simulink model "simu_actuating_fins"  (R2025b)
settings: Solver=FixedStepAuto  StartTime=0.0  StopTime=7  FixedStep=0.01  RelTol=1e-3
model workspace (MAT data in the model file):
  T_data = [16.81; 22.34; 22.23; 21.49; 20; 20.21; 18.09; 15.74; 13.4; 10.85; 10.21; 8.94; 8.83; 8.62; 8.62; 8.62; 8.51; 8.72; 8.51; 8.51; 7.77; 7.02; 5.64; 3.83; 2.23; 0.96; 0]
  aero_data.Alpha = [0; 2; 4]
  aero_data.CD = [0.20580088598; 0.20580088598; 0.20580088598]
  aero_data.CL = [0; 0.0625795358549; 0.124860076206]
  aero_data.CP = [0.999; 0.999; 0.999]
  t_data = [0.01; 0.03; 0.11; 0.26; 0.37; 0.47; 0.67; 0.99; 1.31; 1.81; 2.49; 3.13; 3.6; 4.11; 4.95; 5.45; 5.58; 5.88; 6.22; 6.46; 6.6; 6.71; 6.79; 6.91; 6.95; 7; 7.05]
undefined symbols (not defined in the file): fractalcoef
libraries: mspsensorlib x1, aerolibatmos2 x1, sharedutil x1
settings Model: Creator=arjun  LastModifiedBy=19725

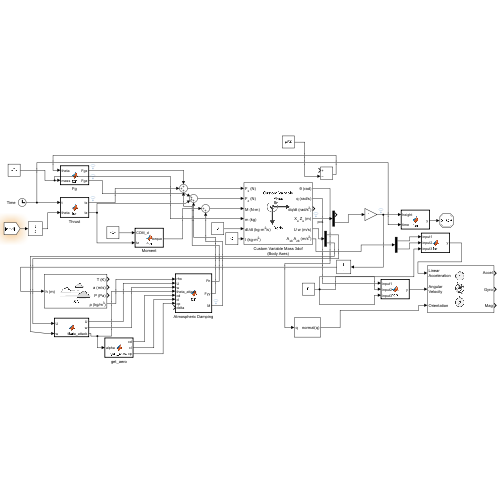
[thumbnail: Simulink's stored preview of the top-level diagram]
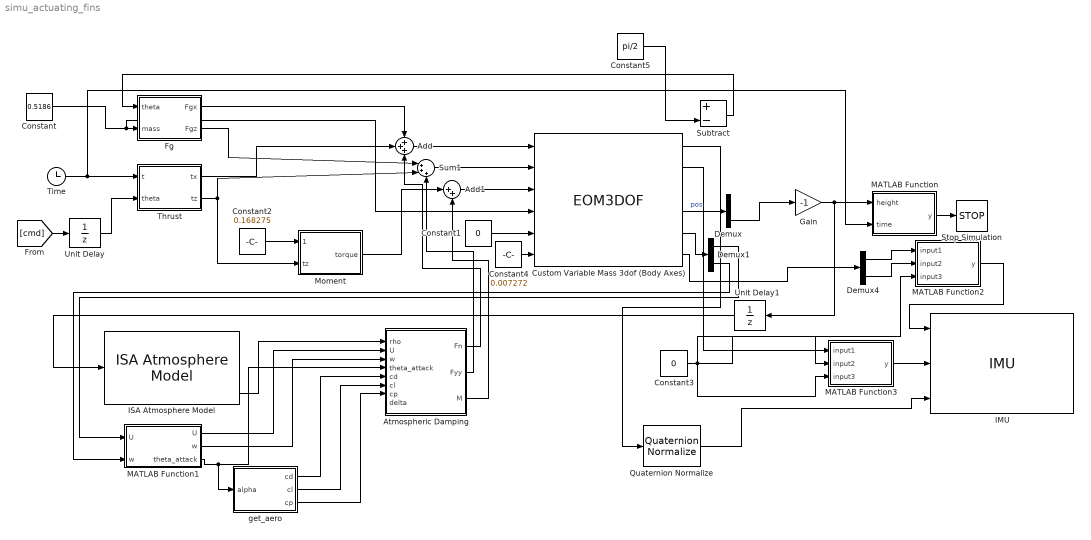
== system simu_actuating_fins ==
  Add : Sum  Inputs=+++
  Add1 : Sum  Inputs=|++
  Atmospheric Damping : MATLAB Function  TreatAsAtomicUnit=on
  Constant : Constant  Value=0.5186
  Constant1 : Constant  Value=0
  Constant2 : Constant  Value=0.168275
  Constant3 : Constant  Value=0
  Constant4 : Constant  Value=0.007272  VectorParams1D=off
  Constant5 : Constant  Value=pi/2
  Custom Variable Mass 3dof (Body Axes) : EOM3DOF  mtype=Custom Variable  theta_ini=deg2rad(93)  g=0
  Demux : Demux  Outputs=2
  Demux1 : Demux  Outputs=2
  Demux4 : Demux  Outputs=2
  Fg : MATLAB Function  TreatAsAtomicUnit=on
  Gain : Gain  Gain=-1
  IMU : mspsensorlib/IMU  DispRefFrame=NED  TemperaturePort=off  Temperature=25  MagneticFieldPort=off  MagneticFieldNED=[ 27.5550, -2.4169, -16.0849 ]  MagneticFieldENU=[ -2.4169, 27.5550, 16.0849 ]  SeedDouble=67  SimulateUsing=Interpreted execution  AccelParamsMeasurementRange=Inf  AccelParamsResolution=0  AccelParamsConstantBias=[ 0, 0, 0 ]  AccelParamsAxesMisalignment=[ 100, 0, 0; 0, 100, 0; 0, 0, 100 ]  AccelParamsNoiseDensity=[ 0, 0, 0 ]  AccelParamsBiasInstability=[ 0, 0, 0 ]  AccelParamsBiasInstabilityNumerator=fractalcoef().Numerator  AccelParamsBiasInstabilityDenominator=fractalcoef().Denominator  AccelParamsRandomWalk=[ 0, 0, 0 ]  AccelParamsNoiseType=double-sided  AccelParamsTemperatureBias=[ 0, 0, 0 ]  AccelParamsTemperatureScaleFactor=[ 0, 0, 0 ]  GyroParamsMeasurementRange=Inf  GyroParamsResolution=0  GyroParamsConstantBias=[ 0, 0, 0 ]  GyroParamsAxesMisalignment=[ 100, 0, 0; 0, 100, 0; 0, 0, 100 ]  GyroParamsAccelerationBias=[ 0, 0, 0 ]  GyroParamsNoiseDensity=[ 0, 0, 0 ]  GyroParamsBiasInstability=[ 0, 0, 0 ]  GyroParamsBiasInstabilityNumerator=fractalcoef().Numerator  GyroParamsBiasInstabilityDenominator=fractalcoef().Denominator  GyroParamsRandomWalk=[ 0, 0, 0 ]  GyroParamsNoiseType=double-sided  GyroParamsTemperatureBias=[ 0, 0, 0 ]  GyroParamsTemperatureScaleFactor=[ 0, 0, 0 ]  MagParamsMeasurementRange=Inf  MagParamsResolution=0  MagParamsConstantBias=[ 0, 0, 0 ]  MagParamsAxesMisalignment=[ 100, 0, 0; 0, 100, 0; 0, 0, 100 ]  MagParamsNoiseDensity=[ 0, 0, 0 ]  MagParamsBiasInstability=[ 0, 0, 0 ]  MagParamsBiasInstabilityNumerator=fractalcoef().Numerator  MagParamsBiasInstabilityDenominator=fractalcoef().Denominator  MagParamsRandomWalk=[ 0, 0, 0 ]  MagParamsNoiseType=double-sided  MagParamsTemperatureBias=[ 0, 0, 0 ]  MagParamsTemperatureScaleFactor=[ 0, 0, 0 ]
  ISA Atmosphere Model : aerolibatmos2/ISA Atmosphere Model  useExtended=off  action=Warning  custom=off  viscosityOut=off  g=9.80665  gamma=1.4  R=287.0531  L=0.0065  h_trop=11000  h_strat=20000  rho0=1.225  P0=101325  T0=288.15  h0=0  S=110.4  Tref=273.15  muref=1.716e-5
  MATLAB Function : MATLAB Function  TreatAsAtomicUnit=on
  MATLAB Function1 : MATLAB Function  TreatAsAtomicUnit=on
  MATLAB Function2 : MATLAB Function  TreatAsAtomicUnit=on
  MATLAB Function3 : MATLAB Function  TreatAsAtomicUnit=on
  Moment : MATLAB Function  TreatAsAtomicUnit=on
  Quaternion Normalize : sharedutil/Quaternion Normalize  aMode=aMode
  Stop Simulation : Stop
  Subtract : Sum  Inputs=+-
  Sum1 : Sum  Inputs=|+++
  Thrust : MATLAB Function  TreatAsAtomicUnit=on
  Time : Clock
  Unit Delay : UnitDelay  SampleTime=-1  HasFrameUpgradeWarning=on
  Unit Delay1 : UnitDelay  SampleTime=-1  HasFrameUpgradeWarning=on
  get_aero : MATLAB Function  TreatAsAtomicUnit=on
  wires:
  Time/1 -> MATLAB Function/2(time), Thrust/1(t)
  Fg/2(Fgz) -> Sum1/1
  Thrust/2(tz) -> Moment/2(tz), Sum1/2
  Sum1/1 -> Custom Variable Mass 3dof (Body Axes)/2
  Add/1 -> Custom Variable Mass 3dof (Body Axes)/1
  Custom Variable Mass 3dof (Body Axes)/4 -> Demux/1  "pos"
  Constant/1 -> Custom Variable Mass 3dof (Body Axes)/4, Fg/2(mass)
  Constant4/1 -> Custom Variable Mass 3dof (Body Axes)/6
  Constant1/1 -> Custom Variable Mass 3dof (Body Axes)/5
  Fg/1(Fgx) -> Add/1
  Thrust/1(tx) -> Add/2
  Constant2/1 -> Moment/1(COM_d)
  Demux/2 -> Gain/1
  MATLAB Function/1(y) -> Stop Simulation/1
  Custom Variable Mass 3dof (Body Axes)/5 -> Demux1/1
  Demux1/1 -> MATLAB Function1/1("U ")
  Demux1/2 -> MATLAB Function1/2("w ")
  MATLAB Function1/1(U) -> Atmospheric Damping/2(U)
  MATLAB Function1/2(w) -> Atmospheric Damping/3(w)
  ISA Atmosphere Model/4 -> Atmospheric Damping/1(rho)
  Moment/1(torque) -> Add1/1
  Add1/1 -> Custom Variable Mass 3dof (Body Axes)/3
  MATLAB Function1/3(theta_attack) -> get_aero/1(alpha), Atmospheric Damping/4(theta_attack)
  get_aero/1(cd) -> Atmospheric Damping/5(cd)
  get_aero/2(cl) -> Atmospheric Damping/6(cl)
  get_aero/3(cp) -> Atmospheric Damping/7(cp)
  Gain/1 -> Unit Delay1/1, MATLAB Function/1(height)
  [cmd] -> Unit Delay/1
  Constant5/1 -> Subtract/2
  Subtract/1 -> Fg/1(theta)
  Unit Delay/1 -> Thrust/2(theta)
  Atmospheric Damping/1(Fn) -> Add/3
  Atmospheric Damping/2(Fyy) -> Sum1/3
  Atmospheric Damping/3(M) -> Add1/2
  Unit Delay1/1 -> ISA Atmosphere Model/1
  MATLAB Function2/1(y) -> IMU/1
  MATLAB Function3/1(y) -> IMU/2
  Demux4/1 -> MATLAB Function2/1(input1)
  Demux4/2 -> MATLAB Function2/2(input2)
  Constant3/1 -> MATLAB Function3/2(input2), MATLAB Function3/3(input3), MATLAB Function2/3(input3)
  Custom Variable Mass 3dof (Body Axes)/6 -> Demux4/1
  Custom Variable Mass 3dof (Body Axes)/2 -> MATLAB Function3/1(input1)
  Custom Variable Mass 3dof (Body Axes)/1 -> Quaternion Normalize/1
  Quaternion Normalize/1 -> IMU/3

== matlab function simu_actuating_fins/Moment ==
  data: COM_d input; torque output; tz input
function torque = fcn(COM_d, tz)

torque = COM_d * tz; % remove

== matlab function simu_actuating_fins/Thrust ==
  data: t input; tx output; tz output; theta input
function [tx, tz] = fcn(t, theta)
    persistent thrust_interp;
    
    if isempty(thrust_interp)
        loadedData = load('interp_thrust_data.mat'); 
        disp(loadedData)
        t_data = loadedData.t_data; 
        T_data = loadedData.T_data; 

        thrust_interp = @(t) interp1(t_data, T_data, t, 'pchip', 'extrap');
    end

    burnout_time = 7.246;
    if t < burnout_time
        T = thrust_interp(t);
    else
        T = 0;
    end

    
    tx = T * cos(theta); % remove
    tz = -T * sin(theta); % remove
end

== matlab function simu_actuating_fins/MATLAB Function ==
  data: height input; time input; y output
function y = fcn(height, time)

if time > 1 && height < 0
    y = 1;
else
    y = 0;
end

== matlab function simu_actuating_fins/Fg ==
  data: theta input; mass input; Fgx output; Fgz output
function [Fgx, Fgz]= fcn(theta, mass)

Fgx = mass * -cos(theta) * 9.8; % potentially remove
Fgz = mass * sin(theta) * -9.8; % potentially remove

== matlab function simu_actuating_fins/MATLAB Function2 ==
  data: y output; input1 input; input2 input; input3 input
function y = fcn(input1, input2, input3)
y = [input1, input2, input3];

== matlab function simu_actuating_fins/MATLAB Function3 ==
  data: y output; input1 input; input2 input; input3 input
function y = fcn(input1, input2, input3)
y = [input1, input2, input3];

== matlab function simu_actuating_fins/MATLAB Function1 ==
  data: U output; w output; U input; w input; theta_attack output
function [U, w, theta_attack] = fcn(U, w)

theta_attack = atan(w/U);

== matlab function simu_actuating_fins/Atmospheric Damping ==
  data: rho input; Fn output; U input; w input; theta_attack input; cd input; cl input; cp input; Fyy output; M output; delta input
function [Fn, Fyy, M] = fcn(rho, U, w, theta_attack, cd, cl, cp, delta)
    V = sqrt(U^2 + w^2); % finding the velocity

    Sref = pi * (0.0762/2)^2; % find the area

    q = 1/2 * rho * V^2; % dynamic pressure (1/2 * air density * velocity squared) 

    alpha = theta_attack;        % assuming theta_attack is angle of attack (rad)

    CL_alpha = 2*pi;             % per rad (thin airfoil theory approximation)
    CL_delta = 0.8;              % control effectiveness (tune this)

    cl = CL_alpha * alpha + CL_delta * delta;

    L = q * cl * Sref; % lift force (multiplies lift coefficient by the area)
    D = q * cd * Sref; % drag force (drag coefficient by the area)

    Xw = -D; % axial wind force
    Zw = -L; % normal wind force
    
    cg = 0.3302; % from nosecone

    Fn =  cos(theta_attack)*Xw - sin(theta_attack)*Zw; % body fixed x-direction forces
    Fyy =  sin(theta_attack)*Xw + cos(theta_attack)*Zw; % body fixed normal momentum
    M = Fyy * (cp - cg); % pitching moment about the center of gravity
end

== matlab function simu_actuating_fins/get_aero ==
  data: alpha input; cd output; cl output; cp output
function [cd, cl, cp] = get_aero(alpha)

    S = load("alpha_interp.mat");  
    Alpha = S.aero_data.Alpha;
    CD_full = S.aero_data.CD;
    CL_full = S.aero_data.CL;
    CP_full = S.aero_data.CP;

    cd = interp1(Alpha, CD_full, alpha, 'linear', 'extrap');
    cl = interp1(Alpha, CL_full, alpha, 'linear', 'extrap');
    cp = interp1(Alpha, CP_full, alpha, 'linear', 'extrap');
    cp = cp * 0.3048;
end
